simulink model "chris_4R_all_primitives"  (R2024b)
settings: Solver=FixedStepDiscrete  StartTime=0.0  StopTime=60  FixedStep=0.1  MaxStep=0.1  RelTol=1e-3
libraries: neural x220, simulink x1, realtime_pacer_lib x1
(part 9 of 9)

== matlab function chris_4R_all_primitives/Jacobians/Cluster Velocities to Cartesian Velocities ==
  data: fwdkin input; xc_err input; x1_err output; yc_err input; th_c_err input; d1_err input; d2_err input; r1_err input; y1_err output; th1_err output; x2_err output; y2_err output; th2_err output; x3_err output; y3_err output; th3_err output; r2_err input; phi_err input; x4_err output; y4_err output; th4_err output
function [x1_err, y1_err, th1_err, x2_err, y2_err, th2_err, x3_err, y3_err, th3_err, x4_err, y4_err, th4_err] = InverseJacobian(fwdkin, xc_err, yc_err, th_c_err, d1_err, d2_err, r1_err, r2_err, phi_err)
% InverseJacobian: Convert parameter errors to corner position/orientation changes
%% Unpacking the information from fwd_kin
d1 = fwdkin(1); % d1 - diagonal 1 length
d2 = fwdkin(2); % d2 - diagonal 2 length
r1 = fwdkin(3); % r1 - intersection ratio 1
r2 = fwdkin(4); % r2 - intersection ratio 2
phi = fwdkin(5); % phi - angle between diagonals
xc = fwdkin(6); % x_c - centroid x
yc = fwdkin(7); % y_c - centroid y
th_c = fwdkin(8); % th_c - overall rotation

%% Inverse Kinematics using Jacobian
% First, compute some common terms used in multiple derivatives
cos_thc = cos(th_c);
sin_thc = sin(th_c);
cos_thc_phi = cos(th_c - phi);
sin_thc_phi = sin(th_c - phi);

% Terms for intersection point derivatives
xi_term1 = d1 * (2*r1 - 1) / 4;
xi_term2 = d2 * (2*r2 - 1) / 4;

%% Partial derivatives for x1
% x1 = x_i - r1 * d1 * cos(th_c)
% where x_i = x_c + (d1 * (2*r1 - 1) * cos(th_c) + d2 * (2*r2 - 1) * cos(th_c - phi)) / 4

% ∂x1/∂xc = 1
dx1_dxc = 1;

% ∂x1/∂yc = 0
dx1_dyc = 0;

% ∂x1/∂th_c = -d1*(2*r1-1)*sin(th_c)/4 - d2*(2*r2-1)*sin(th_c-phi)/4 + r1*d1*sin(th_c)
dx1_dthc = -xi_term1*sin_thc - xi_term2*sin_thc_phi + r1*d1*sin_thc;

% ∂x1/∂d1 = (2*r1-1)*cos(th_c)/4 - r1*cos(th_c)
dx1_dd1 = (2*r1 - 1)*cos_thc/4 - r1*cos_thc;

% ∂x1/∂d2 = (2*r2-1)*cos(th_c-phi)/4
dx1_dd2 = (2*r2 - 1)*cos_thc_phi/4;

% ∂x1/∂r1 = d1*cos(th_c)/2 - d1*cos(th_c)
dx1_dr1 = d1*cos_thc/2 - d1*cos_thc;

% ∂x1/∂r2 = d2*cos(th_c-phi)/2
dx1_dr2 = d2*cos_thc_phi/2;

% ∂x1/∂phi = d2*(2*r2-1)*sin(th_c-phi)/4
dx1_dphi = xi_term2*sin_thc_phi;

% Calculate x1_err
x1_err = dx1_dxc*xc_err + dx1_dyc*yc_err + dx1_dthc*th_c_err + dx1_dd1*d1_err + dx1_dd2*d2_err + dx1_dr1*r1_err + dx1_dr2*r2_err + dx1_dphi*phi_err;

%% Partial derivatives for y1
% y1 = y_i - r1 * d1 * sin(th_c)

% ∂y1/∂xc = 0
dy1_dxc = 0;

% ∂y1/∂yc = 1
dy1_dyc = 1;

% ∂y1/∂th_c = d1*(2*r1-1)*cos(th_c)/4 + d2*(2*r2-1)*cos(th_c-phi)/4 - r1*d1*cos(th_c)
dy1_dthc = xi_term1*cos_thc + xi_term2*cos_thc_phi - r1*d1*cos_thc;

% ∂y1/∂d1 = (2*r1-1)*sin(th_c)/4 - r1*sin(th_c)
dy1_dd1 = (2*r1 - 1)*sin_thc/4 - r1*sin_thc;

% ∂y1/∂d2 = (2*r2-1)*sin(th_c-phi)/4
dy1_dd2 = (2*r2 - 1)*sin_thc_phi/4;

% ∂y1/∂r1 = d1*sin(th_c)/2 - d1*sin(th_c)
dy1_dr1 = d1*sin_thc/2 - d1*sin_thc;

% ∂y1/∂r2 = d2*sin(th_c-phi)/2
dy1_dr2 = d2*sin_thc_phi/2;

% ∂y1/∂phi = -d2*(2*r2-1)*cos(th_c-phi)/4
dy1_dphi = -xi_term2*cos_thc_phi;

% Calculate y1_err
y1_err = dy1_dxc*xc_err + dy1_dyc*yc_err + dy1_dthc*th_c_err + dy1_dd1*d1_err + dy1_dd2*d2_err + dy1_dr1*r1_err + dy1_dr2*r2_err + dy1_dphi*phi_err;

%% Partial derivatives for x2
% x2 = x_i - r2 * d2 * cos(th_c - phi)

% ∂x2/∂xc = 1
dx2_dxc = 1;

% ∂x2/∂yc = 0
dx2_dyc = 0;

% ∂x2/∂th_c = -d1*(2*r1-1)*sin(th_c)/4 - d2*(2*r2-1)*sin(th_c-phi)/4 + r2*d2*sin(th_c-phi)
dx2_dthc = -xi_term1*sin_thc - xi_term2*sin_thc_phi + r2*d2*sin_thc_phi;

% ∂x2/∂d1 = (2*r1-1)*cos(th_c)/4
dx2_dd1 = (2*r1 - 1)*cos_thc/4;

% ∂x2/∂d2 = (2*r2-1)*cos(th_c-phi)/4 - r2*cos(th_c-phi)
dx2_dd2 = (2*r2 - 1)*cos_thc_phi/4 - r2*cos_thc_phi;

% ∂x2/∂r1 = d1*cos(th_c)/2
dx2_dr1 = d1*cos_thc/2;

% ∂x2/∂r2 = d2*cos(th_c-phi)/2 - d2*cos(th_c-phi)
dx2_dr2 = d2*cos_thc_phi/2 - d2*cos_thc_phi;

% ∂x2/∂phi = d2*(2*r2-1)*sin(th_c-phi)/4 - r2*d2*sin(th_c-phi)
dx2_dphi = xi_term2*sin_thc_phi - r2*d2*sin_thc_phi;

% Calculate x2_err
x2_err = dx2_dxc*xc_err + dx2_dyc*yc_err + dx2_dthc*th_c_err + dx2_dd1*d1_err + dx2_dd2*d2_err + dx2_dr1*r1_err + dx2_dr2*r2_err + dx2_dphi*phi_err;

%% Partial derivatives for y2
% y2 = y_i - r2 * d2 * sin(th_c - phi)

% ∂y2/∂xc = 0
dy2_dxc = 0;

% ∂y2/∂yc = 1
dy2_dyc = 1;

% ∂y2/∂th_c = d1*(2*r1-1)*cos(th_c)/4 + d2*(2*r2-1)*cos(th_c-phi)/4 - r2*d2*cos(th_c-phi)
dy2_dthc = xi_term1*cos_thc + xi_term2*cos_thc_phi - r2*d2*cos_thc_phi;

% ∂y2/∂d1 = (2*r1-1)*sin(th_c)/4
dy2_dd1 = (2*r1 - 1)*sin_thc/4;

% ∂y2/∂d2 = (2*r2-1)*sin(th_c-phi)/4 - r2*sin(th_c-phi)
dy2_dd2 = (2*r2 - 1)*sin_thc_phi/4 - r2*sin_thc_phi;

% ∂y2/∂r1 = d1*sin(th_c)/2
dy2_dr1 = d1*sin_thc/2;

% ∂y2/∂r2 = d2*sin(th_c-phi)/2 - d2*sin(th_c-phi)
dy2_dr2 = d2*sin_thc_phi/2 - d2*sin_thc_phi;

% ∂y2/∂phi = -d2*(2*r2-1)*cos(th_c-phi)/4 + r2*d2*cos(th_c-phi)
dy2_dphi = -xi_term2*cos_thc_phi + r2*d2*cos_thc_phi;

% Calculate y2_err
y2_err = dy2_dxc*xc_err + dy2_dyc*yc_err + dy2_dthc*th_c_err + dy2_dd1*d1_err + dy2_dd2*d2_err + dy2_dr1*r1_err + dy2_dr2*r2_err + dy2_dphi*phi_err;

%% Partial derivatives for x3
% x3 = x_i + (1 - r1) * d1 * cos(th_c)

% ∂x3/∂xc = 1
dx3_dxc = 1;

% ∂x3/∂yc = 0
dx3_dyc = 0;

% ∂x3/∂th_c = -d1*(2*r1-1)*sin(th_c)/4 - d2*(2*r2-1)*sin(th_c-phi)/4 - (1-r1)*d1*sin(th_c)
dx3_dthc = -xi_term1*sin_thc - xi_term2*sin_thc_phi - (1-r1)*d1*sin_thc;

% ∂x3/∂d1 = (2*r1-1)*cos(th_c)/4 + (1-r1)*cos(th_c)
dx3_dd1 = (2*r1 - 1)*cos_thc/4 + (1-r1)*cos_thc;

% ∂x3/∂d2 = (2*r2-1)*cos(th_c-phi)/4
dx3_dd2 = (2*r2 - 1)*cos_thc_phi/4;

% ∂x3/∂r1 = d1*cos(th_c)/2 - d1*cos(th_c)
dx3_dr1 = d1*cos_thc/2 - d1*cos_thc;

% ∂x3/∂r2 = d2*cos(th_c-phi)/2
dx3_dr2 = d2*cos_thc_phi/2;

% ∂x3/∂phi = d2*(2*r2-1)*sin(th_c-phi)/4
dx3_dphi = xi_term2*sin_thc_phi;

% Calculate x3_err
x3_err = dx3_dxc*xc_err + dx3_dyc*yc_err + dx3_dthc*th_c_err + dx3_dd1*d1_err + dx3_dd2*d2_err + dx3_dr1*r1_err + dx3_dr2*r2_err + dx3_dphi*phi_err;

%% Partial derivatives for y3
% y3 = y_i + (1 - r1) * d1 * sin(th_c)

% ∂y3/∂xc = 0
dy3_dxc = 0;

% ∂y3/∂yc = 1
dy3_dyc = 1;

% ∂y3/∂th_c = d1*(2*r1-1)*cos(th_c)/4 + d2*(2*r2-1)*cos(th_c-phi)/4 + (1-r1)*d1*cos(th_c)
dy3_dthc = xi_term1*cos_thc + xi_term2*cos_thc_phi + (1-r1)*d1*cos_thc;

% ∂y3/∂d1 = (2*r1-1)*sin(th_c)/4 + (1-r1)*sin(th_c)
dy3_dd1 = (2*r1 - 1)*sin_thc/4 + (1-r1)*sin_thc;

% ∂y3/∂d2 = (2*r2-1)*sin(th_c-phi)/4
dy3_dd2 = (2*r2 - 1)*sin_thc_phi/4;

% ∂y3/∂r1 = d1*sin(th_c)/2 - d1*sin(th_c)
dy3_dr1 = d1*sin_thc/2 - d1*sin_thc;

% ∂y3/∂r2 = d2*sin(th_c-phi)/2
dy3_dr2 = d2*sin_thc_phi/2;

% ∂y3/∂phi = -d2*(2*r2-1)*cos(th_c-phi)/4
dy3_dphi = -xi_term2*cos_thc_phi;

% Calculate y3_err
y3_err = dy3_dxc*xc_err + dy3_dyc*yc_err + dy3_dthc*th_c_err + dy3_dd1*d1_err + dy3_dd2*d2_err + dy3_dr1*r1_err + dy3_dr2*r2_err + dy3_dphi*phi_err;

%% Partial derivatives for x4
% x4 = x_i + (1 - r2) * d2 * cos(th_c - phi)

% ∂x4/∂xc = 1
dx4_dxc = 1;

% ∂x4/∂yc = 0
dx4_dyc = 0;

% ∂x4/∂th_c = -d1*(2*r1-1)*sin(th_c)/4 - d2*(2*r2-1)*sin(th_c-phi)/4 - (1-r2)*d2*sin(th_c-phi)
dx4_dthc = -xi_term1*sin_thc - xi_term2*sin_thc_phi - (1-r2)*d2*sin_thc_phi;

% ∂x4/∂d1 = (2*r1-1)*cos(th_c)/4
dx4_dd1 = (2*r1 - 1)*cos_thc/4;

% ∂x4/∂d2 = (2*r2-1)*cos(th_c-phi)/4 + (1-r2)*cos(th_c-phi)
dx4_dd2 = (2*r2 - 1)*cos_thc_phi/4 + (1-r2)*cos_thc_phi;

% ∂x4/∂r1 = d1*cos(th_c)/2
dx4_dr1 = d1*cos_thc/2;

% ∂x4/∂r2 = d2*cos(th_c-phi)/2 - d2*cos(th_c-phi)
dx4_dr2 = d2*cos_thc_phi/2 - d2*cos_thc_phi;

% ∂x4/∂phi = d2*(2*r2-1)*sin(th_c-phi)/4 + (1-r2)*d2*sin(th_c-phi)
dx4_dphi = xi_term2*sin_thc_phi + (1-r2)*d2*sin_thc_phi;

% Calculate x4_err
x4_err = dx4_dxc*xc_err + dx4_dyc*yc_err + dx4_dthc*th_c_err + dx4_dd1*d1_err + dx4_dd2*d2_err + dx4_dr1*r1_err + dx4_dr2*r2_err + dx4_dphi*phi_err;

%% Partial derivatives for y4
% y4 = y_i + (1 - r2) * d2 * sin(th_c - phi)

% ∂y4/∂xc = 0
dy4_dxc = 0;

% ∂y4/∂yc = 1
dy4_dyc = 1;

% ∂y4/∂th_c = d1*(2*r1-1)*cos(th_c)/4 + d2*(2*r2-1)*cos(th_c-phi)/4 + (1-r2)*d2*cos(th_c-phi)
dy4_dthc = xi_term1*cos_thc + xi_term2*cos_thc_phi + (1-r2)*d2*cos_thc_phi;

% ∂y4/∂d1 = (2*r1-1)*sin(th_c)/4
dy4_dd1 = (2*r1 - 1)*sin_thc/4;

% ∂y4/∂d2 = (2*r2-1)*sin(th_c-phi)/4 + (1-r2)*sin(th_c-phi)
dy4_dd2 = (2*r2 - 1)*sin_thc_phi/4 + (1-r2)*sin_thc_phi;

% ∂y4/∂r1 = d1*sin(th_c)/2
dy4_dr1 = d1*sin_thc/2;

% ∂y4/∂r2 = d2*sin(th_c-phi)/2 - d2*sin(th_c-phi)
dy4_dr2 = d2*sin_thc_phi/2 - d2*sin_thc_phi;

% ∂y4/∂phi = -d2*(2*r2-1)*cos(th_c-phi)/4 - (1-r2)*d2*cos(th_c-phi)
dy4_dphi = -xi_term2*cos_thc_phi - (1-r2)*d2*cos_thc_phi;

% Calculate y4_err
y4_err = dy4_dxc*xc_err + dy4_dyc*yc_err + dy4_dthc*th_c_err + dy4_dd1*d1_err + dy4_dd2*d2_err + dy4_dr1*r1_err + dy4_dr2*r2_err + dy4_dphi*phi_err;

%% Orientation changes
% th1, th2, th3, th4 represent deviation from overall rotation thc
% Assigning Th1 values of 0.
th1_err = 0; % Corner 1 orientation deviation from thc
th2_err = 0; % Corner 2 orientation deviation from thc
th3_err = 0; % Corner 3 orientation deviation from thc
th4_err = 0; % Corner 4 orientation deviation from thc

end

== matlab function chris_4R_all_primitives/Jacobians/Critical_point_predicter/MATLAB Function ==
  data: x output; x1 input; y output; y1 input; u1 input; v1 input; x2 input; y2 input; u2 input; v2 input; x3 input; y3 input; u3 input; v3 input; x4 input; y4 input; u4 input; v4 input
function [x, y] = Criticalpointfinder(x1, y1, u1, v1, x2, y2, u2, v2, x3, y3, u3, v3, x4, y4, u4, v4)
% Given 4 points in a 2D Vector Field,
% Use two combinations of 3 points to determine critical points,
% then average the results.
% For a 2D vector field, we can represent it as:
% u = |a b| |x| + |c|
% v = |d e| |y| + |f|

% First computation using points 1, 2, 3
A_123 = [x1 y1 1;
         x2 y2 1;
         x3 y3 1];
         
b_u_123 = [u1; u2; u3];
b_v_123 = [v1; v2; v3];

% Solve for coefficients (exactly determined system)
u_coeffs_123 = A_123\b_u_123; % [a; b; c]
v_coeffs_123 = A_123\b_v_123; % [d; e; f]

% Extract Jacobian matrix for first set
J_123 = [u_coeffs_123(1) u_coeffs_123(2);
         v_coeffs_123(1) v_coeffs_123(2)]; % [a b; d e]

% Extract constant terms for first set
K_123 = [-u_coeffs_123(3); -v_coeffs_123(3)]; % [-c; -f]

% Solve for first critical point
if abs(det(J_123)) < 1e-10
    x_123 = NaN;
    y_123 = NaN;
    warning('First Jacobian (points 1,2,3) is singular. No unique critical point.');
else
    solution_123 = J_123\K_123;
    x_123 = solution_123(1);
    y_123 = solution_123(2);
end

% Second computation using points 1, 3, 4
A_134 = [x1 y1 1;
         x3 y3 1;
         x4 y4 1];
         
b_u_134 = [u1; u3; u4];
b_v_134 = [v1; v3; v4];

% Solve for coefficients (exactly determined system)
u_coeffs_134 = A_134\b_u_134; % [a; b; c]
v_coeffs_134 = A_134\b_v_134; % [d; e; f]

% Extract Jacobian matrix for second set
J_134 = [u_coeffs_134(1) u_coeffs_134(2);
         v_coeffs_134(1) v_coeffs_134(2)]; % [a b; d e]

% Extract constant terms for second set
K_134 = [-u_coeffs_134(3); -v_coeffs_134(3)]; % [-c; -f]

% Solve for second critical point
if abs(det(J_134)) < 1e-10
    x_134 = NaN;
    y_134 = NaN;
    warning('Second Jacobian (points 1,3,4) is singular. No unique critical point.');
else
    solution_134 = J_134\K_134;
    x_134 = solution_134(1);
    y_134 = solution_134(2);
end

% Average the two results
if isnan(x_123) || isnan(y_123)
    % If first computation failed, use only the second
    x = x_134;
    y = y_134;
elseif isnan(x_134) || isnan(y_134)
    % If second computation failed, use only the first
    x = x_123;
    y = y_123;
else
    % Both computations succeeded, average them
    x = (x_123 + x_134) / 2;
    y = (y_123 + y_134) / 2;
    %x = (x_134 + x_134) / 2;
    %y = (y_134 + y_134) / 2;
end

% Optional: Display individual results for debugging
if nargout == 0 || true % You can set this to false to suppress output
    fprintf('Critical point from points 1,2,3: (%.6f, %.6f)\n', x_123, y_123);
    fprintf('Critical point from points 1,3,4: (%.6f, %.6f)\n', x_134, y_134);
    fprintf('Averaged critical point: (%.6f, %.6f)\n', x, y);
end

end

== matlab function chris_4R_all_primitives/Robot_signal_processing_2/Global to Body Rotation Matrix ==
  data: u input; y output
function y = fcn(u)

y = [cos(u) -sin(u) 0; sin(u) cos(u) 0; 0 0 1];

== matlab function chris_4R_all_primitives/Jacobian/Cartesian to Cluster Variables ==
  data: fwdkin output; x1 input; x_c output; y1 input; th1 input; x2 input; y2 input; th2 input; x3 input; y3 input; th3 input; y_c output; th_c output; d1 output; d2 output; r1 output; x4 input; y4 input; r2 output; phi output; th4 input
function [fwdkin, x_c, y_c, th_c, d1, d2, r1, r2, phi] = Forward_Kinematics(x1, y1, th1, x2, y2, th2, x3, y3, th3, x4, y4, th4)
% Forward_Kinematics: Convert corner coordinates to diagonal parameters
% 
% Inputs:
%   x1, y1, th1: Position and orientation of corner 1
%   x2, y2, th2: Position and orientation of corner 2  
%   x3, y3, th3: Position and orientation of corner 3
%   x4, y4, th4: Position and orientation of corner 4
%
% Outputs:
%   fwdkin: [d1, d2, r1, r2, phi, x_c, y_c, th_c] - diagonal parameters
%   x_c, y_c: Centroid coordinates
%   th_c: Overall rotation angle (theta)
%   d1, d2: Diagonal lengths
%   r1, r2: Intersection ratios
%   theta_1: Same as th_c (for compatibility)

% Centre frame (centroid)
x_c = (x1 + x2 + x3 + x4) / 4;
y_c = (y1 + y2 + y3 + y4) / 4;

% Diagonal lengths
d1 = sqrt((x3 - x1)^2 + (y3 - y1)^2);  % Diagonal 1-3
d2 = sqrt((x4 - x2)^2 + (y4 - y2)^2);  % Diagonal 2-4

% Overall rotation angle (angle of diagonal 1-3)
th_c = atan2(y3 - y1, x3 - x1);

% Angle between diagonals
phi = -atan2(y4 - y2, x4 - x2) + atan2(y3 - y1, x3 - x1);

% Intersection ratios using line intersection method
% Solving for where diagonals 1-3 and 2-4 intersect
delta = (x3 - x1) * (y2 - y4) + (y3 - y1) * (x4 - x2);


% Standard intersection calculation
r1 = ((x2 - x1) * (y2 - y4) + (y2 - y1) * (x4 - x2)) / delta;
r2 = ((x3 - x1) * (y2 - y1) - (y3 - y1) * (x2 - x1)) / delta;


% Combining all readings into fwdkin vector
fwdkin = [0 0 0 0 0 0 0 0];
fwdkin(1) = d1;      % Diagonal 1 length
fwdkin(2) = d2;      % Diagonal 2 length  
fwdkin(3) = r1;      % Intersection ratio 1
fwdkin(4) = r2;      % Intersection ratio 2
fwdkin(5) = phi;     % Angle between diagonals
fwdkin(6) = x_c;     % Centroid x
fwdkin(7) = y_c;     % Centroid y
fwdkin(8) = th_c;    % Overall rotation angle

end

== matlab function chris_4R_all_primitives/Jacobian/Cluster Velocities to Cartesian Velocities ==
  data: fwdkin input; xc_err input; x1_err output; yc_err input; th_c_err input; d1_err input; d2_err input; r1_err input; y1_err output; th1_err output; x2_err output; y2_err output; th2_err output; x3_err output; y3_err output; th3_err output; r2_err input; phi_err input; x4_err output; y4_err output; th4_err output
function [x1_err, y1_err, th1_err, x2_err, y2_err, th2_err, x3_err, y3_err, th3_err, x4_err, y4_err, th4_err] = InverseJacobian(fwdkin, xc_err, yc_err, th_c_err, d1_err, d2_err, r1_err, r2_err, phi_err)
% InverseJacobian: Convert parameter errors to corner position/orientation changes
%% Unpacking the information from fwd_kin
d1 = fwdkin(1); % d1 - diagonal 1 length
d2 = fwdkin(2); % d2 - diagonal 2 length
r1 = fwdkin(3); % r1 - intersection ratio 1
r2 = fwdkin(4); % r2 - intersection ratio 2
phi = fwdkin(5); % phi - angle between diagonals
xc = fwdkin(6); % x_c - centroid x
yc = fwdkin(7); % y_c - centroid y
th_c = fwdkin(8); % th_c - overall rotation

%% Inverse Kinematics using Jacobian
% First, compute some common terms used in multiple derivatives
cos_thc = cos(th_c);
sin_thc = sin(th_c);
cos_thc_phi = cos(th_c - phi);
sin_thc_phi = sin(th_c - phi);

% Terms for intersection point derivatives
xi_term1 = d1 * (2*r1 - 1) / 4;
xi_term2 = d2 * (2*r2 - 1) / 4;

%% Partial derivatives for x1
% x1 = x_i - r1 * d1 * cos(th_c)
% where x_i = x_c + (d1 * (2*r1 - 1) * cos(th_c) + d2 * (2*r2 - 1) * cos(th_c - phi)) / 4

% ∂x1/∂xc = 1
dx1_dxc = 1;

% ∂x1/∂yc = 0
dx1_dyc = 0;

% ∂x1/∂th_c = -d1*(2*r1-1)*sin(th_c)/4 - d2*(2*r2-1)*sin(th_c-phi)/4 + r1*d1*sin(th_c)
dx1_dthc = -xi_term1*sin_thc - xi_term2*sin_thc_phi + r1*d1*sin_thc;

% ∂x1/∂d1 = (2*r1-1)*cos(th_c)/4 - r1*cos(th_c)
dx1_dd1 = (2*r1 - 1)*cos_thc/4 - r1*cos_thc;

% ∂x1/∂d2 = (2*r2-1)*cos(th_c-phi)/4
dx1_dd2 = (2*r2 - 1)*cos_thc_phi/4;

% ∂x1/∂r1 = d1*cos(th_c)/2 - d1*cos(th_c)
dx1_dr1 = d1*cos_thc/2 - d1*cos_thc;

% ∂x1/∂r2 = d2*cos(th_c-phi)/2
dx1_dr2 = d2*cos_thc_phi/2;

% ∂x1/∂phi = d2*(2*r2-1)*sin(th_c-phi)/4
dx1_dphi = xi_term2*sin_thc_phi;

% Calculate x1_err
x1_err = dx1_dxc*xc_err + dx1_dyc*yc_err + dx1_dthc*th_c_err + dx1_dd1*d1_err + dx1_dd2*d2_err + dx1_dr1*r1_err + dx1_dr2*r2_err + dx1_dphi*phi_err;

%% Partial derivatives for y1
% y1 = y_i - r1 * d1 * sin(th_c)

% ∂y1/∂xc = 0
dy1_dxc = 0;

% ∂y1/∂yc = 1
dy1_dyc = 1;

% ∂y1/∂th_c = d1*(2*r1-1)*cos(th_c)/4 + d2*(2*r2-1)*cos(th_c-phi)/4 - r1*d1*cos(th_c)
dy1_dthc = xi_term1*cos_thc + xi_term2*cos_thc_phi - r1*d1*cos_thc;

% ∂y1/∂d1 = (2*r1-1)*sin(th_c)/4 - r1*sin(th_c)
dy1_dd1 = (2*r1 - 1)*sin_thc/4 - r1*sin_thc;

% ∂y1/∂d2 = (2*r2-1)*sin(th_c-phi)/4
dy1_dd2 = (2*r2 - 1)*sin_thc_phi/4;

% ∂y1/∂r1 = d1*sin(th_c)/2 - d1*sin(th_c)
dy1_dr1 = d1*sin_thc/2 - d1*sin_thc;

% ∂y1/∂r2 = d2*sin(th_c-phi)/2
dy1_dr2 = d2*sin_thc_phi/2;

% ∂y1/∂phi = -d2*(2*r2-1)*cos(th_c-phi)/4
dy1_dphi = -xi_term2*cos_thc_phi;

% Calculate y1_err
y1_err = dy1_dxc*xc_err + dy1_dyc*yc_err + dy1_dthc*th_c_err + dy1_dd1*d1_err + dy1_dd2*d2_err + dy1_dr1*r1_err + dy1_dr2*r2_err + dy1_dphi*phi_err;

%% Partial derivatives for x2
% x2 = x_i - r2 * d2 * cos(th_c - phi)

% ∂x2/∂xc = 1
dx2_dxc = 1;

% ∂x2/∂yc = 0
dx2_dyc = 0;

% ∂x2/∂th_c = -d1*(2*r1-1)*sin(th_c)/4 - d2*(2*r2-1)*sin(th_c-phi)/4 + r2*d2*sin(th_c-phi)
dx2_dthc = -xi_term1*sin_thc - xi_term2*sin_thc_phi + r2*d2*sin_thc_phi;

% ∂x2/∂d1 = (2*r1-1)*cos(th_c)/4
dx2_dd1 = (2*r1 - 1)*cos_thc/4;

% ∂x2/∂d2 = (2*r2-1)*cos(th_c-phi)/4 - r2*cos(th_c-phi)
dx2_dd2 = (2*r2 - 1)*cos_thc_phi/4 - r2*cos_thc_phi;

% ∂x2/∂r1 = d1*cos(th_c)/2
dx2_dr1 = d1*cos_thc/2;

% ∂x2/∂r2 = d2*cos(th_c-phi)/2 - d2*cos(th_c-phi)
dx2_dr2 = d2*cos_thc_phi/2 - d2*cos_thc_phi;

% ∂x2/∂phi = d2*(2*r2-1)*sin(th_c-phi)/4 - r2*d2*sin(th_c-phi)
dx2_dphi = xi_term2*sin_thc_phi - r2*d2*sin_thc_phi;

% Calculate x2_err
x2_err = dx2_dxc*xc_err + dx2_dyc*yc_err + dx2_dthc*th_c_err + dx2_dd1*d1_err + dx2_dd2*d2_err + dx2_dr1*r1_err + dx2_dr2*r2_err + dx2_dphi*phi_err;

%% Partial derivatives for y2
% y2 = y_i - r2 * d2 * sin(th_c - phi)

% ∂y2/∂xc = 0
dy2_dxc = 0;

% ∂y2/∂yc = 1
dy2_dyc = 1;

% ∂y2/∂th_c = d1*(2*r1-1)*cos(th_c)/4 + d2*(2*r2-1)*cos(th_c-phi)/4 - r2*d2*cos(th_c-phi)
dy2_dthc = xi_term1*cos_thc + xi_term2*cos_thc_phi - r2*d2*cos_thc_phi;

% ∂y2/∂d1 = (2*r1-1)*sin(th_c)/4
dy2_dd1 = (2*r1 - 1)*sin_thc/4;

% ∂y2/∂d2 = (2*r2-1)*sin(th_c-phi)/4 - r2*sin(th_c-phi)
dy2_dd2 = (2*r2 - 1)*sin_thc_phi/4 - r2*sin_thc_phi;

% ∂y2/∂r1 = d1*sin(th_c)/2
dy2_dr1 = d1*sin_thc/2;

% ∂y2/∂r2 = d2*sin(th_c-phi)/2 - d2*sin(th_c-phi)
dy2_dr2 = d2*sin_thc_phi/2 - d2*sin_thc_phi;

% ∂y2/∂phi = -d2*(2*r2-1)*cos(th_c-phi)/4 + r2*d2*cos(th_c-phi)
dy2_dphi = -xi_term2*cos_thc_phi + r2*d2*cos_thc_phi;

% Calculate y2_err
y2_err = dy2_dxc*xc_err + dy2_dyc*yc_err + dy2_dthc*th_c_err + dy2_dd1*d1_err + dy2_dd2*d2_err + dy2_dr1*r1_err + dy2_dr2*r2_err + dy2_dphi*phi_err;

%% Partial derivatives for x3
% x3 = x_i + (1 - r1) * d1 * cos(th_c)

% ∂x3/∂xc = 1
dx3_dxc = 1;

% ∂x3/∂yc = 0
dx3_dyc = 0;

% ∂x3/∂th_c = -d1*(2*r1-1)*sin(th_c)/4 - d2*(2*r2-1)*sin(th_c-phi)/4 - (1-r1)*d1*sin(th_c)
dx3_dthc = -xi_term1*sin_thc - xi_term2*sin_thc_phi - (1-r1)*d1*sin_thc;

% ∂x3/∂d1 = (2*r1-1)*cos(th_c)/4 + (1-r1)*cos(th_c)
dx3_dd1 = (2*r1 - 1)*cos_thc/4 + (1-r1)*cos_thc;

% ∂x3/∂d2 = (2*r2-1)*cos(th_c-phi)/4
dx3_dd2 = (2*r2 - 1)*cos_thc_phi/4;

% ∂x3/∂r1 = d1*cos(th_c)/2 - d1*cos(th_c)
dx3_dr1 = d1*cos_thc/2 - d1*cos_thc;

% ∂x3/∂r2 = d2*cos(th_c-phi)/2
dx3_dr2 = d2*cos_thc_phi/2;

% ∂x3/∂phi = d2*(2*r2-1)*sin(th_c-phi)/4
dx3_dphi = xi_term2*sin_thc_phi;

% Calculate x3_err
x3_err = dx3_dxc*xc_err + dx3_dyc*yc_err + dx3_dthc*th_c_err + dx3_dd1*d1_err + dx3_dd2*d2_err + dx3_dr1*r1_err + dx3_dr2*r2_err + dx3_dphi*phi_err;

%% Partial derivatives for y3
% y3 = y_i + (1 - r1) * d1 * sin(th_c)

% ∂y3/∂xc = 0
dy3_dxc = 0;

% ∂y3/∂yc = 1
dy3_dyc = 1;

% ∂y3/∂th_c = d1*(2*r1-1)*cos(th_c)/4 + d2*(2*r2-1)*cos(th_c-phi)/4 + (1-r1)*d1*cos(th_c)
dy3_dthc = xi_term1*cos_thc + xi_term2*cos_thc_phi + (1-r1)*d1*cos_thc;

% ∂y3/∂d1 = (2*r1-1)*sin(th_c)/4 + (1-r1)*sin(th_c)
dy3_dd1 = (2*r1 - 1)*sin_thc/4 + (1-r1)*sin_thc;

% ∂y3/∂d2 = (2*r2-1)*sin(th_c-phi)/4
dy3_dd2 = (2*r2 - 1)*sin_thc_phi/4;

% ∂y3/∂r1 = d1*sin(th_c)/2 - d1*sin(th_c)
dy3_dr1 = d1*sin_thc/2 - d1*sin_thc;

% ∂y3/∂r2 = d2*sin(th_c-phi)/2
dy3_dr2 = d2*sin_thc_phi/2;

% ∂y3/∂phi = -d2*(2*r2-1)*cos(th_c-phi)/4
dy3_dphi = -xi_term2*cos_thc_phi;

% Calculate y3_err
y3_err = dy3_dxc*xc_err + dy3_dyc*yc_err + dy3_dthc*th_c_err + dy3_dd1*d1_err + dy3_dd2*d2_err + dy3_dr1*r1_err + dy3_dr2*r2_err + dy3_dphi*phi_err;

%% Partial derivatives for x4
% x4 = x_i + (1 - r2) * d2 * cos(th_c - phi)

% ∂x4/∂xc = 1
dx4_dxc = 1;

% ∂x4/∂yc = 0
dx4_dyc = 0;

% ∂x4/∂th_c = -d1*(2*r1-1)*sin(th_c)/4 - d2*(2*r2-1)*sin(th_c-phi)/4 - (1-r2)*d2*sin(th_c-phi)
dx4_dthc = -xi_term1*sin_thc - xi_term2*sin_thc_phi - (1-r2)*d2*sin_thc_phi;

% ∂x4/∂d1 = (2*r1-1)*cos(th_c)/4
dx4_dd1 = (2*r1 - 1)*cos_thc/4;

% ∂x4/∂d2 = (2*r2-1)*cos(th_c-phi)/4 + (1-r2)*cos(th_c-phi)
dx4_dd2 = (2*r2 - 1)*cos_thc_phi/4 + (1-r2)*cos_thc_phi;

% ∂x4/∂r1 = d1*cos(th_c)/2
dx4_dr1 = d1*cos_thc/2;

% ∂x4/∂r2 = d2*cos(th_c-phi)/2 - d2*cos(th_c-phi)
dx4_dr2 = d2*cos_thc_phi/2 - d2*cos_thc_phi;

% ∂x4/∂phi = d2*(2*r2-1)*sin(th_c-phi)/4 + (1-r2)*d2*sin(th_c-phi)
dx4_dphi = xi_term2*sin_thc_phi + (1-r2)*d2*sin_thc_phi;

% Calculate x4_err
x4_err = dx4_dxc*xc_err + dx4_dyc*yc_err + dx4_dthc*th_c_err + dx4_dd1*d1_err + dx4_dd2*d2_err + dx4_dr1*r1_err + dx4_dr2*r2_err + dx4_dphi*phi_err;

%% Partial derivatives for y4
% y4 = y_i + (1 - r2) * d2 * sin(th_c - phi)

% ∂y4/∂xc = 0
dy4_dxc = 0;

% ∂y4/∂yc = 1
dy4_dyc = 1;

% ∂y4/∂th_c = d1*(2*r1-1)*cos(th_c)/4 + d2*(2*r2-1)*cos(th_c-phi)/4 + (1-r2)*d2*cos(th_c-phi)
dy4_dthc = xi_term1*cos_thc + xi_term2*cos_thc_phi + (1-r2)*d2*cos_thc_phi;

% ∂y4/∂d1 = (2*r1-1)*sin(th_c)/4
dy4_dd1 = (2*r1 - 1)*sin_thc/4;

% ∂y4/∂d2 = (2*r2-1)*sin(th_c-phi)/4 + (1-r2)*sin(th_c-phi)
dy4_dd2 = (2*r2 - 1)*sin_thc_phi/4 + (1-r2)*sin_thc_phi;

% ∂y4/∂r1 = d1*sin(th_c)/2
dy4_dr1 = d1*sin_thc/2;

% ∂y4/∂r2 = d2*sin(th_c-phi)/2 - d2*sin(th_c-phi)
dy4_dr2 = d2*sin_thc_phi/2 - d2*sin_thc_phi;

% ∂y4/∂phi = -d2*(2*r2-1)*cos(th_c-phi)/4 - (1-r2)*d2*cos(th_c-phi)
dy4_dphi = -xi_term2*cos_thc_phi - (1-r2)*d2*cos_thc_phi;

% Calculate y4_err
y4_err = dy4_dxc*xc_err + dy4_dyc*yc_err + dy4_dthc*th_c_err + dy4_dd1*d1_err + dy4_dd2*d2_err + dy4_dr1*r1_err + dy4_dr2*r2_err + dy4_dphi*phi_err;

%% Orientation changes
% th1, th2, th3, th4 represent deviation from overall rotation thc
% Assigning Th1 values of 0.
th1_err = 0; % Corner 1 orientation deviation from thc
th2_err = 0; % Corner 2 orientation deviation from thc
th3_err = 0; % Corner 3 orientation deviation from thc
th4_err = 0; % Corner 4 orientation deviation from thc

end

== matlab function chris_4R_all_primitives/Jacobian/MATLAB Function ==
  data: xc_velocity output; xc_actual input; yc_velocity output; yc_actual input; x_critical_point input; y_critical_point input; clockwise input; desired_radius input
function [xc_velocity, yc_velocity] = Orbiter(xc_actual, yc_actual, x_critical_point, y_critical_point, clockwise, desired_radius)


% Setting some gains
K_p = 0.1; % Proportional gain for radius control
orbit_speed = 0.15; % Base orbital speed

% Calculate vector from actual position to critical point
dx = x_critical_point - xc_actual;
dy = y_critical_point - yc_actual;

% Calculate current distance (radius) from critical point
current_radius = sqrt(dx^2 + dy^2);


% Create unit vector pointing from actual position to critical point
unit_x = dx / current_radius;
unit_y = dy / current_radius;

% Create unit vector for orbital motion (tangential)
% For clockwise rotation (+1): [x, y] -> [y, -x]
% For counterclockwise rotation (-1): [x, y] -> [-y, x]
orbit_x = clockwise * unit_y;
orbit_y = -clockwise * unit_x;

% Calculate radius error (positive when too close, negative when too far)
radius_error = desired_radius - current_radius;

% Calculate radial velocity component - negative when need to move outward, positive when need to move inward
radial_adjustment = K_p * radius_error;

% Apply adjustments:
% 1. Base orbital motion (tangential)
% 2. Radial adjustment (inward/outward)
xc_velocity = orbit_speed * orbit_x - radial_adjustment * unit_x;
yc_velocity = orbit_speed * orbit_y - radial_adjustment * unit_y;
xc_velocity = xc_velocity;
yc_velocity = yc_velocity;
end

== matlab function chris_4R_all_primitives/Robot_signal_processing_3/Global to Body Rotation Matrix ==
  data: u input; y output
function y = fcn(u)

y = [cos(u) -sin(u) 0; sin(u) cos(u) 0; 0 0 1];

== matlab function chris_4R_all_primitives/Jacobian/Critical_point_predicter/MATLAB Function ==
  data: x output; x1 input; y output; y1 input; u1 input; v1 input; x2 input; y2 input; u2 input; v2 input; x3 input; y3 input; u3 input; v3 input; x4 input; y4 input; u4 input; v4 input
function [x, y] = Criticalpointfinder(x1, y1, u1, v1, x2, y2, u2, v2, x3, y3, u3, v3, x4, y4, u4, v4)
% Given 4 points in a 2D Vector Field,
% Determine the Jacobian using least squares,
% then Determine the critical points.
% For a 2D vector field, we can represent it as:
% u = |a b| |x| + |c|
% v = |d e| |y| + |f|

% Set up matrices for overdetermined system (4 equations, 3 unknowns)
A = [x1 y1 1; 
     x2 y2 1; 
     x3 y3 1;
     x4 y4 1];
     
b_u = [u1; u2; u3; u4];
b_v = [v1; v2; v3; v4];

% Solve for coefficients using least squares (A'*A*x = A'*b)
% This finds the best fit when the system is overdetermined
u_coeffs = A\b_u; % [a; b; c] - MATLAB automatically uses least squares for overdetermined systems
v_coeffs = A\b_v; % [d; e; f]

% Alternative explicit least squares solution (same result):
% u_coeffs = (A'*A)\(A'*b_u);
% v_coeffs = (A'*A)\(A'*b_v);

% Extract Jacobian matrix
J = [u_coeffs(1) u_coeffs(2); 
     v_coeffs(1) v_coeffs(2)]; % [a b; d e]

% Extract constant terms
K = [-u_coeffs(3); -v_coeffs(3)]; % [-c; -f]

% Solve for critical point (where u = 0 and v = 0)
% This gives us: J*[x; y] = K
if abs(det(J)) < 1e-10 % Check if determinant is close to zero
    x = NaN;
    y = NaN;
    warning('Jacobian is singular or near-singular. No unique critical point exists.');
else
    solution = J\K;
    x = solution(1);
    y = solution(2);
    fprintf('Critical point from all 4 points 1,2,3: (%.6f, %.6f)\n', x, y)
end

% Optional: Calculate residuals to check quality of fit
if nargout > 2
    % Calculate predicted velocities at the 4 points
    u_pred = A * u_coeffs;
    v_pred = A * v_coeffs;
    
    % Calculate residuals
    u_residuals = b_u - u_pred;
    v_residuals = b_v - v_pred;
    
    % Root mean square error
    rmse_u = sqrt(mean(u_residuals.^2));
    rmse_v = sqrt(mean(v_residuals.^2));
    
    fprintf('Fit quality:\n');
    fprintf('  RMSE for u: %.6f\n', rmse_u);
    fprintf('  RMSE for v: %.6f\n', rmse_v);
end

end

== matlab function chris_4R_all_primitives/Jacobians/MATLAB Function ==
  data: xc_velocity output; xc_actual input; yc_velocity output; yc_actual input; x_critical_point input; y_critical_point input; clockwise input; desired_radius input
function [xc_velocity, yc_velocity] = Orbiter(xc_actual, yc_actual, x_critical_point, y_critical_point, clockwise, desired_radius)


% Setting some gains
K_p = 0.1; % Proportional gain for radius control
orbit_speed = 0.15; % Base orbital speed

% Calculate vector from actual position to critical point
dx = x_critical_point - xc_actual;
dy = y_critical_point - yc_actual;

% Calculate current distance (radius) from critical point
current_radius = sqrt(dx^2 + dy^2);


% Create unit vector pointing from actual position to critical point
unit_x = dx / current_radius;
unit_y = dy / current_radius;

% Create unit vector for orbital motion (tangential)
% For clockwise rotation (+1): [x, y] -> [y, -x]
% For counterclockwise rotation (-1): [x, y] -> [-y, x]
orbit_x = clockwise * unit_y;
orbit_y = -clockwise * unit_x;

% Calculate radius error (positive when too close, negative when too far)
radius_error = desired_radius - current_radius;

% Calculate radial velocity component - negative when need to move outward, positive when need to move inward
radial_adjustment = K_p * radius_error;

% Apply adjustments:
% 1. Base orbital motion (tangential)
% 2. Radial adjustment (inward/outward)
xc_velocity = orbit_speed * orbit_x - radial_adjustment * unit_x;
yc_velocity = orbit_speed * orbit_y - radial_adjustment * unit_y;
xc_velocity = xc_velocity;
yc_velocity = yc_velocity;
end

== matlab function chris_4R_all_primitives/Jacobians/Cartesian to Cluster Variables1 ==
  data: angle output; thc_error output; xc_actual input; yc_actual input; thc_actual input; xc_desired input; yc_desired input
function [angle, thc_error] = Theta_controller(xc_actual, yc_actual, thc_actual, xc_desired, yc_desired)
    % Calculate the angle of the line from actual to desired position
    angle = atan2(yc_desired - yc_actual, xc_desired - xc_actual);
    
    % Normalize thc_actual to [-pi, pi] 
    thc_actual_wrapped = atan2(sin(thc_actual), cos(thc_actual));
    
    % Calculate error and wrap it
    thc_error = angle - thc_actual_wrapped;
    thc_error = 2*atan2(sin(thc_error), cos(thc_error));
end

== matlab function chris_4R_all_primitives/Cluster_Controller_setpoint/Cartesian to Cluster Variables ==
  data: fwdkin output; x1 input; x_c output; y1 input; th1 input; x2 input; y2 input; th2 input; x3 input; y3 input; th3 input; y_c output; th_c output; d1 output; d2 output; r1 output; x4 input; y4 input; r2 output; phi output; th4 input
function [fwdkin, x_c, y_c, th_c, d1, d2, r1, r2, phi] = Forward_Kinematics(x1, y1, th1, x2, y2, th2, x3, y3, th3, x4, y4, th4)
% Forward_Kinematics: Convert corner coordinates to diagonal parameters
% 
% Inputs:
%   x1, y1, th1: Position and orientation of corner 1
%   x2, y2, th2: Position and orientation of corner 2  
%   x3, y3, th3: Position and orientation of corner 3
%   x4, y4, th4: Position and orientation of corner 4
%
% Outputs:
%   fwdkin: [d1, d2, r1, r2, phi, x_c, y_c, th_c] - diagonal parameters
%   x_c, y_c: Centroid coordinates
%   th_c: Overall rotation angle (theta)
%   d1, d2: Diagonal lengths
%   r1, r2: Intersection ratios
%   theta_1: Same as th_c (for compatibility)

% Centre frame (centroid)
x_c = (x1 + x2 + x3 + x4) / 4;
y_c = (y1 + y2 + y3 + y4) / 4;

% Diagonal lengths
d1 = sqrt((x3 - x1)^2 + (y3 - y1)^2);  % Diagonal 1-3
d2 = sqrt((x4 - x2)^2 + (y4 - y2)^2);  % Diagonal 2-4

% Overall rotation angle (angle of diagonal 1-3)
th_c = atan2(y3 - y1, x3 - x1);

% Angle between diagonals
phi = -atan2(y4 - y2, x4 - x2) + atan2(y3 - y1, x3 - x1);

% Intersection ratios using line intersection method
% Solving for where diagonals 1-3 and 2-4 intersect
delta = (x3 - x1) * (y2 - y4) + (y3 - y1) * (x4 - x2);


% Standard intersection calculation
r1 = ((x2 - x1) * (y2 - y4) + (y2 - y1) * (x4 - x2)) / delta;
r2 = ((x3 - x1) * (y2 - y1) - (y3 - y1) * (x2 - x1)) / delta;


% Combining all readings into fwdkin vector
fwdkin = [0 0 0 0 0 0 0 0];
fwdkin(1) = d1;      % Diagonal 1 length
fwdkin(2) = d2;      % Diagonal 2 length  
fwdkin(3) = r1;      % Intersection ratio 1
fwdkin(4) = r2;      % Intersection ratio 2
fwdkin(5) = phi;     % Angle between diagonals
fwdkin(6) = x_c;     % Centroid x
fwdkin(7) = y_c;     % Centroid y
fwdkin(8) = th_c;    % Overall rotation angle

end

== matlab function chris_4R_all_primitives/Cluster_Controller_setpoint/Cluster Velocities to Cartesian Velocities ==
  data: fwdkin input; xc_err input; x1_err output; yc_err input; th_c_err input; d1_err input; d2_err input; r1_err input; y1_err output; th1_err output; x2_err output; y2_err output; th2_err output; x3_err output; y3_err output; th3_err output; r2_err input; phi_err input; x4_err output; y4_err output; th4_err output
function [x1_err, y1_err, th1_err, x2_err, y2_err, th2_err, x3_err, y3_err, th3_err, x4_err, y4_err, th4_err] = InverseJacobian(fwdkin, xc_err, yc_err, th_c_err, d1_err, d2_err, r1_err, r2_err, phi_err)
% InverseJacobian: Convert parameter errors to corner position/orientation changes
%% Unpacking the information from fwd_kin
d1 = fwdkin(1); % d1 - diagonal 1 length
d2 = fwdkin(2); % d2 - diagonal 2 length
r1 = fwdkin(3); % r1 - intersection ratio 1
r2 = fwdkin(4); % r2 - intersection ratio 2
phi = fwdkin(5); % phi - angle between diagonals
xc = fwdkin(6); % x_c - centroid x
yc = fwdkin(7); % y_c - centroid y
th_c = fwdkin(8); % th_c - overall rotation

%% Inverse Kinematics using Jacobian
% First, compute some common terms used in multiple derivatives
cos_thc = cos(th_c);
sin_thc = sin(th_c);
cos_thc_phi = cos(th_c - phi);
sin_thc_phi = sin(th_c - phi);

% Terms for intersection point derivatives
xi_term1 = d1 * (2*r1 - 1) / 4;
xi_term2 = d2 * (2*r2 - 1) / 4;

%% Partial derivatives for x1
% x1 = x_i - r1 * d1 * cos(th_c)
% where x_i = x_c + (d1 * (2*r1 - 1) * cos(th_c) + d2 * (2*r2 - 1) * cos(th_c - phi)) / 4

% ∂x1/∂xc = 1
dx1_dxc = 1;

% ∂x1/∂yc = 0
dx1_dyc = 0;

% ∂x1/∂th_c = -d1*(2*r1-1)*sin(th_c)/4 - d2*(2*r2-1)*sin(th_c-phi)/4 + r1*d1*sin(th_c)
dx1_dthc = -xi_term1*sin_thc - xi_term2*sin_thc_phi + r1*d1*sin_thc;

% ∂x1/∂d1 = (2*r1-1)*cos(th_c)/4 - r1*cos(th_c)
dx1_dd1 = (2*r1 - 1)*cos_thc/4 - r1*cos_thc;

% ∂x1/∂d2 = (2*r2-1)*cos(th_c-phi)/4
dx1_dd2 = (2*r2 - 1)*cos_thc_phi/4;

% ∂x1/∂r1 = d1*cos(th_c)/2 - d1*cos(th_c)
dx1_dr1 = d1*cos_thc/2 - d1*cos_thc;

% ∂x1/∂r2 = d2*cos(th_c-phi)/2
dx1_dr2 = d2*cos_thc_phi/2;

% ∂x1/∂phi = d2*(2*r2-1)*sin(th_c-phi)/4
dx1_dphi = xi_term2*sin_thc_phi;

% Calculate x1_err
x1_err = dx1_dxc*xc_err + dx1_dyc*yc_err + dx1_dthc*th_c_err + dx1_dd1*d1_err + dx1_dd2*d2_err + dx1_dr1*r1_err + dx1_dr2*r2_err + dx1_dphi*phi_err;

%% Partial derivatives for y1
% y1 = y_i - r1 * d1 * sin(th_c)

% ∂y1/∂xc = 0
dy1_dxc = 0;

% ∂y1/∂yc = 1
dy1_dyc = 1;

% ∂y1/∂th_c = d1*(2*r1-1)*cos(th_c)/4 + d2*(2*r2-1)*cos(th_c-phi)/4 - r1*d1*cos(th_c)
dy1_dthc = xi_term1*cos_thc + xi_term2*cos_thc_phi - r1*d1*cos_thc;

% ∂y1/∂d1 = (2*r1-1)*sin(th_c)/4 - r1*sin(th_c)
dy1_dd1 = (2*r1 - 1)*sin_thc/4 - r1*sin_thc;

% ∂y1/∂d2 = (2*r2-1)*sin(th_c-phi)/4
dy1_dd2 = (2*r2 - 1)*sin_thc_phi/4;

% ∂y1/∂r1 = d1*sin(th_c)/2 - d1*sin(th_c)
dy1_dr1 = d1*sin_thc/2 - d1*sin_thc;

% ∂y1/∂r2 = d2*sin(th_c-phi)/2
dy1_dr2 = d2*sin_thc_phi/2;

% ∂y1/∂phi = -d2*(2*r2-1)*cos(th_c-phi)/4
dy1_dphi = -xi_term2*cos_thc_phi;

% Calculate y1_err
y1_err = dy1_dxc*xc_err + dy1_dyc*yc_err + dy1_dthc*th_c_err + dy1_dd1*d1_err + dy1_dd2*d2_err + dy1_dr1*r1_err + dy1_dr2*r2_err + dy1_dphi*phi_err;

%% Partial derivatives for x2
% x2 = x_i - r2 * d2 * cos(th_c - phi)

% ∂x2/∂xc = 1
dx2_dxc = 1;

% ∂x2/∂yc = 0
dx2_dyc = 0;

% ∂x2/∂th_c = -d1*(2*r1-1)*sin(th_c)/4 - d2*(2*r2-1)*sin(th_c-phi)/4 + r2*d2*sin(th_c-phi)
dx2_dthc = -xi_term1*sin_thc - xi_term2*sin_thc_phi + r2*d2*sin_thc_phi;

% ∂x2/∂d1 = (2*r1-1)*cos(th_c)/4
dx2_dd1 = (2*r1 - 1)*cos_thc/4;

% ∂x2/∂d2 = (2*r2-1)*cos(th_c-phi)/4 - r2*cos(th_c-phi)
dx2_dd2 = (2*r2 - 1)*cos_thc_phi/4 - r2*cos_thc_phi;

% ∂x2/∂r1 = d1*cos(th_c)/2
dx2_dr1 = d1*cos_thc/2;

% ∂x2/∂r2 = d2*cos(th_c-phi)/2 - d2*cos(th_c-phi)
dx2_dr2 = d2*cos_thc_phi/2 - d2*cos_thc_phi;

% ∂x2/∂phi = d2*(2*r2-1)*sin(th_c-phi)/4 - r2*d2*sin(th_c-phi)
dx2_dphi = xi_term2*sin_thc_phi - r2*d2*sin_thc_phi;

% Calculate x2_err
x2_err = dx2_dxc*xc_err + dx2_dyc*yc_err + dx2_dthc*th_c_err + dx2_dd1*d1_err + dx2_dd2*d2_err + dx2_dr1*r1_err + dx2_dr2*r2_err + dx2_dphi*phi_err;

%% Partial derivatives for y2
% y2 = y_i - r2 * d2 * sin(th_c - phi)

% ∂y2/∂xc = 0
dy2_dxc = 0;

% ∂y2/∂yc = 1
dy2_dyc = 1;

% ∂y2/∂th_c = d1*(2*r1-1)*cos(th_c)/4 + d2*(2*r2-1)*cos(th_c-phi)/4 - r2*d2*cos(th_c-phi)
dy2_dthc = xi_term1*cos_thc + xi_term2*cos_thc_phi - r2*d2*cos_thc_phi;

% ∂y2/∂d1 = (2*r1-1)*sin(th_c)/4
dy2_dd1 = (2*r1 - 1)*sin_thc/4;

% ∂y2/∂d2 = (2*r2-1)*sin(th_c-phi)/4 - r2*sin(th_c-phi)
dy2_dd2 = (2*r2 - 1)*sin_thc_phi/4 - r2*sin_thc_phi;

% ∂y2/∂r1 = d1*sin(th_c)/2
dy2_dr1 = d1*sin_thc/2;

% ∂y2/∂r2 = d2*sin(th_c-phi)/2 - d2*sin(th_c-phi)
dy2_dr2 = d2*sin_thc_phi/2 - d2*sin_thc_phi;

% ∂y2/∂phi = -d2*(2*r2-1)*cos(th_c-phi)/4 + r2*d2*cos(th_c-phi)
dy2_dphi = -xi_term2*cos_thc_phi + r2*d2*cos_thc_phi;

% Calculate y2_err
y2_err = dy2_dxc*xc_err + dy2_dyc*yc_err + dy2_dthc*th_c_err + dy2_dd1*d1_err + dy2_dd2*d2_err + dy2_dr1*r1_err + dy2_dr2*r2_err + dy2_dphi*phi_err;

%% Partial derivatives for x3
% x3 = x_i + (1 - r1) * d1 * cos(th_c)

% ∂x3/∂xc = 1
dx3_dxc = 1;

% ∂x3/∂yc = 0
dx3_dyc = 0;

% ∂x3/∂th_c = -d1*(2*r1-1)*sin(th_c)/4 - d2*(2*r2-1)*sin(th_c-phi)/4 - (1-r1)*d1*sin(th_c)
dx3_dthc = -xi_term1*sin_thc - xi_term2*sin_thc_phi - (1-r1)*d1*sin_thc;

% ∂x3/∂d1 = (2*r1-1)*cos(th_c)/4 + (1-r1)*cos(th_c)
dx3_dd1 = (2*r1 - 1)*cos_thc/4 + (1-r1)*cos_thc;

% ∂x3/∂d2 = (2*r2-1)*cos(th_c-phi)/4
dx3_dd2 = (2*r2 - 1)*cos_thc_phi/4;

% ∂x3/∂r1 = d1*cos(th_c)/2 - d1*cos(th_c)
dx3_dr1 = d1*cos_thc/2 - d1*cos_thc;

% ∂x3/∂r2 = d2*cos(th_c-phi)/2
dx3_dr2 = d2*cos_thc_phi/2;

% ∂x3/∂phi = d2*(2*r2-1)*sin(th_c-phi)/4
dx3_dphi = xi_term2*sin_thc_phi;

% Calculate x3_err
x3_err = dx3_dxc*xc_err + dx3_dyc*yc_err + dx3_dthc*th_c_err + dx3_dd1*d1_err + dx3_dd2*d2_err + dx3_dr1*r1_err + dx3_dr2*r2_err + dx3_dphi*phi_err;

%% Partial derivatives for y3
% y3 = y_i + (1 - r1) * d1 * sin(th_c)

% ∂y3/∂xc = 0
dy3_dxc = 0;

% ∂y3/∂yc = 1
dy3_dyc = 1;

% ∂y3/∂th_c = d1*(2*r1-1)*cos(th_c)/4 + d2*(2*r2-1)*cos(th_c-phi)/4 + (1-r1)*d1*cos(th_c)
dy3_dthc = xi_term1*cos_thc + xi_term2*cos_thc_phi + (1-r1)*d1*cos_thc;

% ∂y3/∂d1 = (2*r1-1)*sin(th_c)/4 + (1-r1)*sin(th_c)
dy3_dd1 = (2*r1 - 1)*sin_thc/4 + (1-r1)*sin_thc;

% ∂y3/∂d2 = (2*r2-1)*sin(th_c-phi)/4
dy3_dd2 = (2*r2 - 1)*sin_thc_phi/4;

% ∂y3/∂r1 = d1*sin(th_c)/2 - d1*sin(th_c)
dy3_dr1 = d1*sin_thc/2 - d1*sin_thc;

% ∂y3/∂r2 = d2*sin(th_c-phi)/2
dy3_dr2 = d2*sin_thc_phi/2;

% ∂y3/∂phi = -d2*(2*r2-1)*cos(th_c-phi)/4
dy3_dphi = -xi_term2*cos_thc_phi;

% Calculate y3_err
y3_err = dy3_dxc*xc_err + dy3_dyc*yc_err + dy3_dthc*th_c_err + dy3_dd1*d1_err + dy3_dd2*d2_err + dy3_dr1*r1_err + dy3_dr2*r2_err + dy3_dphi*phi_err;

%% Partial derivatives for x4
% x4 = x_i + (1 - r2) * d2 * cos(th_c - phi)

% ∂x4/∂xc = 1
dx4_dxc = 1;

% ∂x4/∂yc = 0
dx4_dyc = 0;

% ∂x4/∂th_c = -d1*(2*r1-1)*sin(th_c)/4 - d2*(2*r2-1)*sin(th_c-phi)/4 - (1-r2)*d2*sin(th_c-phi)
dx4_dthc = -xi_term1*sin_thc - xi_term2*sin_thc_phi - (1-r2)*d2*sin_thc_phi;

% ∂x4/∂d1 = (2*r1-1)*cos(th_c)/4
dx4_dd1 = (2*r1 - 1)*cos_thc/4;

% ∂x4/∂d2 = (2*r2-1)*cos(th_c-phi)/4 + (1-r2)*cos(th_c-phi)
dx4_dd2 = (2*r2 - 1)*cos_thc_phi/4 + (1-r2)*cos_thc_phi;

% ∂x4/∂r1 = d1*cos(th_c)/2
dx4_dr1 = d1*cos_thc/2;

% ∂x4/∂r2 = d2*cos(th_c-phi)/2 - d2*cos(th_c-phi)
dx4_dr2 = d2*cos_thc_phi/2 - d2*cos_thc_phi;

% ∂x4/∂phi = d2*(2*r2-1)*sin(th_c-phi)/4 + (1-r2)*d2*sin(th_c-phi)
dx4_dphi = xi_term2*sin_thc_phi + (1-r2)*d2*sin_thc_phi;

% Calculate x4_err
x4_err = dx4_dxc*xc_err + dx4_dyc*yc_err + dx4_dthc*th_c_err + dx4_dd1*d1_err + dx4_dd2*d2_err + dx4_dr1*r1_err + dx4_dr2*r2_err + dx4_dphi*phi_err;

%% Partial derivatives for y4
% y4 = y_i + (1 - r2) * d2 * sin(th_c - phi)

% ∂y4/∂xc = 0
dy4_dxc = 0;

% ∂y4/∂yc = 1
dy4_dyc = 1;

% ∂y4/∂th_c = d1*(2*r1-1)*cos(th_c)/4 + d2*(2*r2-1)*cos(th_c-phi)/4 + (1-r2)*d2*cos(th_c-phi)
dy4_dthc = xi_term1*cos_thc + xi_term2*cos_thc_phi + (1-r2)*d2*cos_thc_phi;

% ∂y4/∂d1 = (2*r1-1)*sin(th_c)/4
dy4_dd1 = (2*r1 - 1)*sin_thc/4;

% ∂y4/∂d2 = (2*r2-1)*sin(th_c-phi)/4 + (1-r2)*sin(th_c-phi)
dy4_dd2 = (2*r2 - 1)*sin_thc_phi/4 + (1-r2)*sin_thc_phi;

% ∂y4/∂r1 = d1*sin(th_c)/2
dy4_dr1 = d1*sin_thc/2;

% ∂y4/∂r2 = d2*sin(th_c-phi)/2 - d2*sin(th_c-phi)
dy4_dr2 = d2*sin_thc_phi/2 - d2*sin_thc_phi;

% ∂y4/∂phi = -d2*(2*r2-1)*cos(th_c-phi)/4 - (1-r2)*d2*cos(th_c-phi)
dy4_dphi = -xi_term2*cos_thc_phi - (1-r2)*d2*cos_thc_phi;

% Calculate y4_err
y4_err = dy4_dxc*xc_err + dy4_dyc*yc_err + dy4_dthc*th_c_err + dy4_dd1*d1_err + dy4_dd2*d2_err + dy4_dr1*r1_err + dy4_dr2*r2_err + dy4_dphi*phi_err;

%% Orientation changes
% th1, th2, th3, th4 represent deviation from overall rotation thc
% Assigning Th1 values of 0.
th1_err = 0; % Corner 1 orientation deviation from thc
th2_err = 0; % Corner 2 orientation deviation from thc
th3_err = 0; % Corner 3 orientation deviation from thc
th4_err = 0; % Corner 4 orientation deviation from thc

end

== matlab function chris_4R_all_primitives/Robot_signal_processing_1/Global to Body Rotation Matrix ==
  data: u input; y output
function y = fcn(u)

y = [cos(u) -sin(u) 0; sin(u) cos(u) 0; 0 0 1];
